simulink model "Async3bitsUpDownCounter"  (R2025b)
settings: Solver=VariableStepAuto  StartTime=0.0  StopTime=Inf  RelTol=1e-3
settings Model: PacingRate=3  Creator=Soochan Kim  LastModifiedBy=Soochan Kim

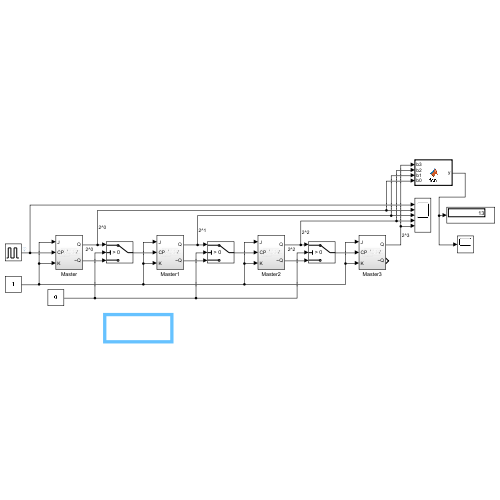
[thumbnail: Simulink's stored preview of the top-level diagram]
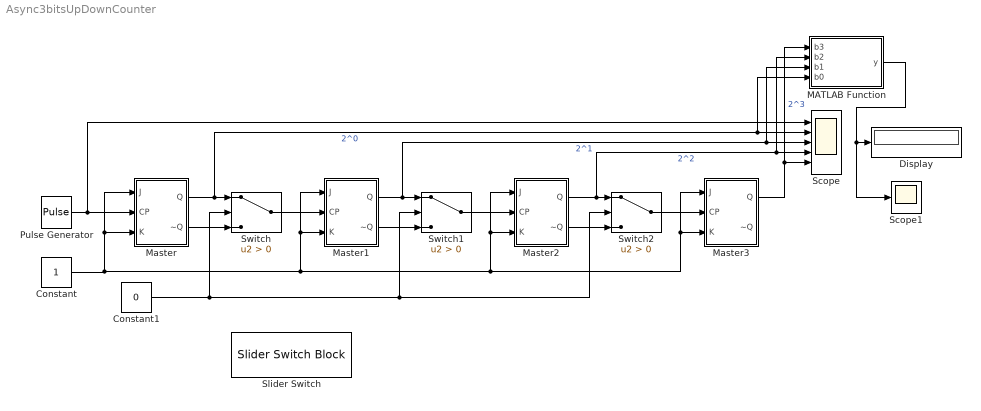
== system Async3bitsUpDownCounter ==
  Constant : Constant
  Constant1 : Constant  Value=0
  Display : Display
  MATLAB Function : MATLAB Function  TreatAsAtomicUnit=on
  Master : Subsystem
  Master1 : Subsystem
  Master2 : Subsystem
  Master3 : Subsystem
  Pulse Generator : DiscretePulseGenerator  PulseType=Time based  Period=1  PulseWidth=50  PhaseDelay=0.5
  Scope : Scope  NumInputPorts=5
      settings: ActiveDisplayYMinimum=-0.12499999999999997  ActiveDisplayYMaximum=1.125
  Scope1 : Scope
      settings: ActiveDisplayYMinimum=-1.8749999999999996  ActiveDisplayYMaximum=16.875
  Slider Switch : SliderSwitchBlock
  Switch : Switch  Criteria=u2 > Threshold  SaturateOnIntegerOverflow=off  InputSameDT=off
  Switch1 : Switch  Criteria=u2 > Threshold  SaturateOnIntegerOverflow=off  InputSameDT=off
  Switch2 : Switch  Criteria=u2 > Threshold  SaturateOnIntegerOverflow=off  InputSameDT=off
  wires:
  Pulse Generator/1 -> Scope/1, Master/2(CP)
  Master/1(Q) -> MATLAB Function/4(b0), Scope/2, Switch/1  "2^0"
  MATLAB Function/1(y) -> Scope1/1, Display/1
  Master/2(~Q) -> Switch/3
  Switch/1 -> Master1/2(CP)
  Switch1/1 -> Master2/2(CP)
  Master1/1(Q) -> MATLAB Function/3(b1), Scope/3, Switch1/1  "2^1"
  Master1/2(~Q) -> Switch1/3
  Master2/1(Q) -> Switch2/1, MATLAB Function/2(b2), Scope/4  "2^2"
  Switch2/1 -> Master3/2(CP)
  Constant/1 -> Master/1(J), Master/3(K), Master3/1(J), Master3/3(K), Master2/1(J), Master2/3(K), Master1/1(J), Master1/3(K)
  Master2/2(~Q) -> Switch2/3
  Constant1/1 -> Switch2/2, Switch1/2, Switch/2
  Master3/1(Q) -> Scope/5, MATLAB Function/1(b3)  "2^3"

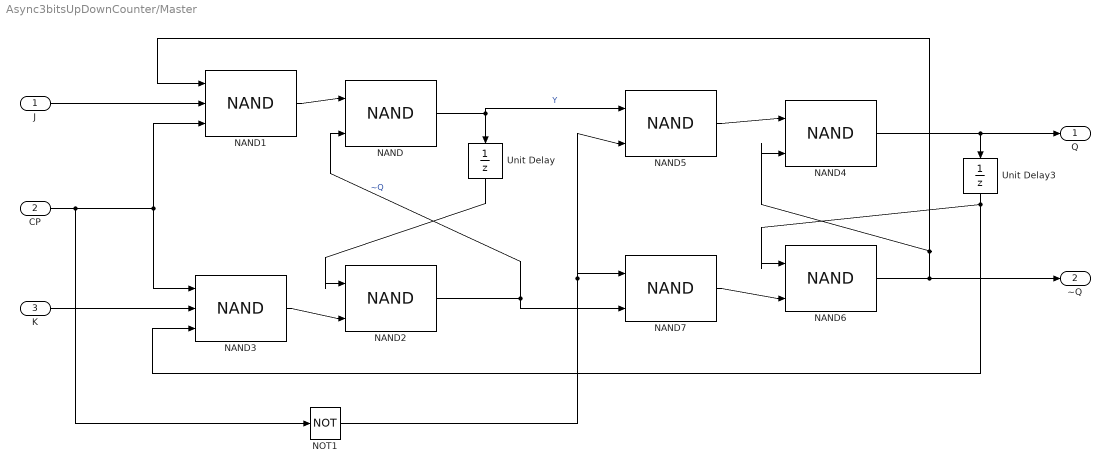
== system Async3bitsUpDownCounter/Master ==
  J : Inport
  CP : Inport  Port=2
  K : Inport  Port=3
  NAND{,2,4..7} (6 alike) : Logic  Operator=NAND  IconShape=distinctive  AllPortsSameDT=off  OutDataTypeStr=boolean
  NAND1 : Logic  Operator=NAND  Inputs=3  IconShape=distinctive  AllPortsSameDT=off  OutDataTypeStr=boolean
  NAND3 : Logic  Operator=NAND  Inputs=3  IconShape=distinctive  AllPortsSameDT=off  OutDataTypeStr=boolean
  NOT1 : Logic  Operator=NOT  IconShape=distinctive  AllPortsSameDT=off  OutDataTypeStr=boolean
  Unit Delay : UnitDelay  SampleTime=0.001  HasFrameUpgradeWarning=on
  Unit Delay3 : UnitDelay  SampleTime=-1  HasFrameUpgradeWarning=on
  Q : Outport
  ~Q : Outport  Port=2
  wires:
  NAND/1 -> Unit Delay/1, NAND5/1  "Y"
  NAND2/1 -> NAND/2, NAND7/2  "~Q"
  Unit Delay/1 -> NAND2/1
  K/1 -> NAND3/2
  NAND1/1 -> NAND/1
  NAND3/1 -> NAND2/2
  J/1 -> NAND1/2
  NAND6/1 -> ~Q/1, NAND1/1, NAND4/2
  Unit Delay3/1 -> NAND3/3, NAND6/1
  NAND5/1 -> NAND4/1
  NAND7/1 -> NAND6/2
  NAND4/1 -> Q/1, Unit Delay3/1
  CP/1 -> NAND1/3, NAND3/1, NOT1/1
  NOT1/1 -> NAND5/2, NAND7/1

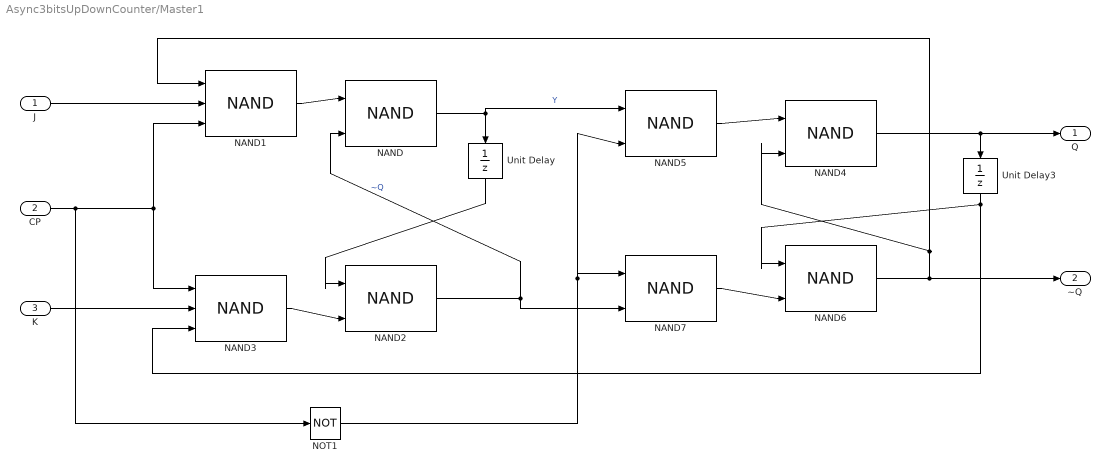
== system Async3bitsUpDownCounter/Master1 ==
  J : Inport
  CP : Inport  Port=2
  K : Inport  Port=3
  NAND{,2,4..7} (6 alike) : Logic  Operator=NAND  IconShape=distinctive  AllPortsSameDT=off  OutDataTypeStr=boolean
  NAND1 : Logic  Operator=NAND  Inputs=3  IconShape=distinctive  AllPortsSameDT=off  OutDataTypeStr=boolean
  NAND3 : Logic  Operator=NAND  Inputs=3  IconShape=distinctive  AllPortsSameDT=off  OutDataTypeStr=boolean
  NOT1 : Logic  Operator=NOT  IconShape=distinctive  AllPortsSameDT=off  OutDataTypeStr=boolean
  Unit Delay : UnitDelay  SampleTime=0.001  HasFrameUpgradeWarning=on
  Unit Delay3 : UnitDelay  SampleTime=-1  HasFrameUpgradeWarning=on
  Q : Outport
  ~Q : Outport  Port=2
  wires:
  NAND/1 -> Unit Delay/1, NAND5/1  "Y"
  NAND2/1 -> NAND/2, NAND7/2  "~Q"
  Unit Delay/1 -> NAND2/1
  K/1 -> NAND3/2
  NAND1/1 -> NAND/1
  NAND3/1 -> NAND2/2
  J/1 -> NAND1/2
  NAND6/1 -> ~Q/1, NAND1/1, NAND4/2
  Unit Delay3/1 -> NAND3/3, NAND6/1
  NAND5/1 -> NAND4/1
  NAND7/1 -> NAND6/2
  NAND4/1 -> Q/1, Unit Delay3/1
  CP/1 -> NAND1/3, NAND3/1, NOT1/1
  NOT1/1 -> NAND5/2, NAND7/1

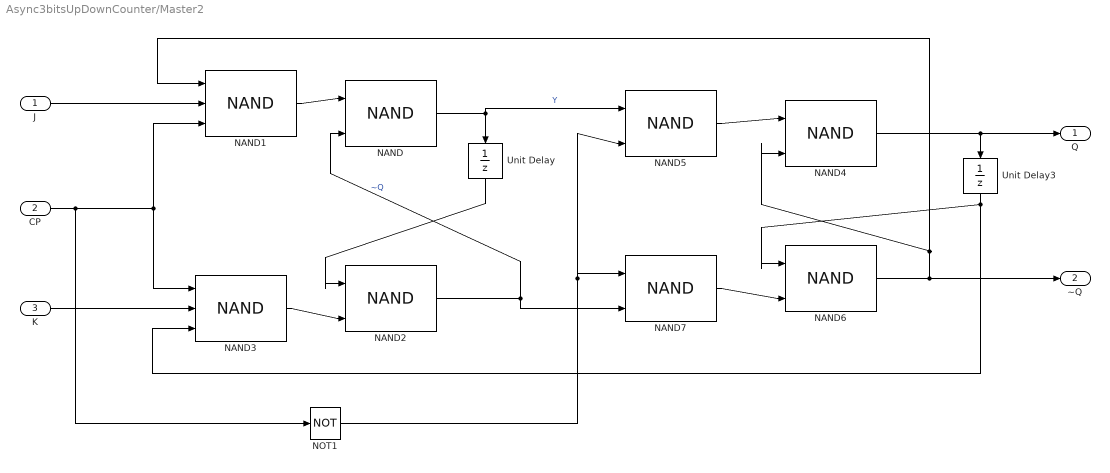
== system Async3bitsUpDownCounter/Master2 ==
  J : Inport
  CP : Inport  Port=2
  K : Inport  Port=3
  NAND{,2,4..7} (6 alike) : Logic  Operator=NAND  IconShape=distinctive  AllPortsSameDT=off  OutDataTypeStr=boolean
  NAND1 : Logic  Operator=NAND  Inputs=3  IconShape=distinctive  AllPortsSameDT=off  OutDataTypeStr=boolean
  NAND3 : Logic  Operator=NAND  Inputs=3  IconShape=distinctive  AllPortsSameDT=off  OutDataTypeStr=boolean
  NOT1 : Logic  Operator=NOT  IconShape=distinctive  AllPortsSameDT=off  OutDataTypeStr=boolean
  Unit Delay : UnitDelay  SampleTime=0.001  HasFrameUpgradeWarning=on
  Unit Delay3 : UnitDelay  SampleTime=-1  HasFrameUpgradeWarning=on
  Q : Outport
  ~Q : Outport  Port=2
  wires:
  NAND/1 -> Unit Delay/1, NAND5/1  "Y"
  NAND2/1 -> NAND/2, NAND7/2  "~Q"
  Unit Delay/1 -> NAND2/1
  K/1 -> NAND3/2
  NAND1/1 -> NAND/1
  NAND3/1 -> NAND2/2
  J/1 -> NAND1/2
  NAND6/1 -> ~Q/1, NAND1/1, NAND4/2
  Unit Delay3/1 -> NAND3/3, NAND6/1
  NAND5/1 -> NAND4/1
  NAND7/1 -> NAND6/2
  NAND4/1 -> Q/1, Unit Delay3/1
  CP/1 -> NAND1/3, NAND3/1, NOT1/1
  NOT1/1 -> NAND5/2, NAND7/1

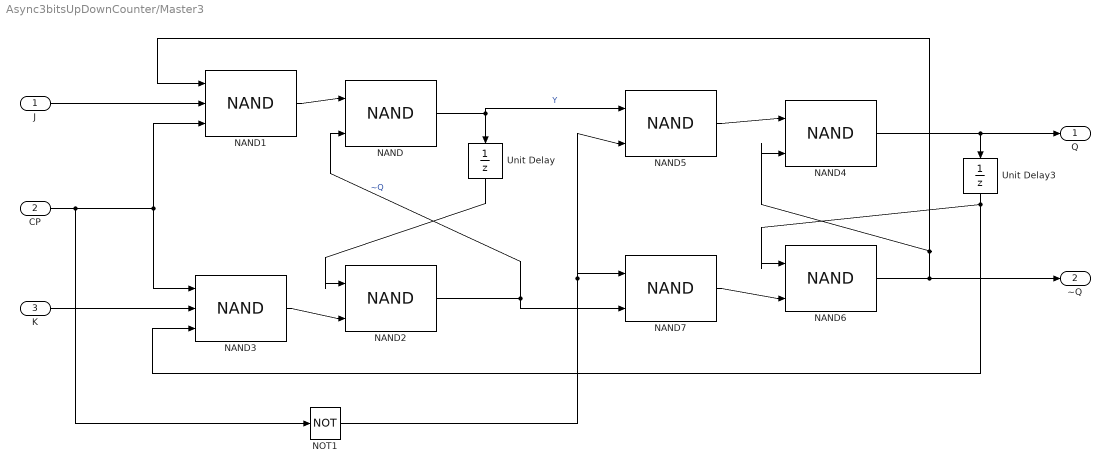
== system Async3bitsUpDownCounter/Master3 ==
  J : Inport
  CP : Inport  Port=2
  K : Inport  Port=3
  NAND{,2,4..7} (6 alike) : Logic  Operator=NAND  IconShape=distinctive  AllPortsSameDT=off  OutDataTypeStr=boolean
  NAND1 : Logic  Operator=NAND  Inputs=3  IconShape=distinctive  AllPortsSameDT=off  OutDataTypeStr=boolean
  NAND3 : Logic  Operator=NAND  Inputs=3  IconShape=distinctive  AllPortsSameDT=off  OutDataTypeStr=boolean
  NOT1 : Logic  Operator=NOT  IconShape=distinctive  AllPortsSameDT=off  OutDataTypeStr=boolean
  Unit Delay : UnitDelay  SampleTime=0.001  HasFrameUpgradeWarning=on
  Unit Delay3 : UnitDelay  SampleTime=-1  HasFrameUpgradeWarning=on
  Q : Outport
  ~Q : Outport  Port=2
  wires:
  NAND/1 -> Unit Delay/1, NAND5/1  "Y"
  NAND2/1 -> NAND/2, NAND7/2  "~Q"
  Unit Delay/1 -> NAND2/1
  K/1 -> NAND3/2
  NAND1/1 -> NAND/1
  NAND3/1 -> NAND2/2
  J/1 -> NAND1/2
  NAND6/1 -> ~Q/1, NAND1/1, NAND4/2
  Unit Delay3/1 -> NAND3/3, NAND6/1
  NAND5/1 -> NAND4/1
  NAND7/1 -> NAND6/2
  NAND4/1 -> Q/1, Unit Delay3/1
  CP/1 -> NAND1/3, NAND3/1, NOT1/1
  NOT1/1 -> NAND5/2, NAND7/1

== matlab function Async3bitsUpDownCounter/MATLAB Function ==
  data: b3 input; b2 input; y output; b1 input; b0 input
function y = fcn(b3, b2, b1, b0)
u = b3*2^3 + b2*2^2 + b1*2^1 + b0

y = u;
